simulink model "parallelizationTest"  (R2017a)
settings: Solver=FixedStepAuto  StartTime=0.0  StopTime=10  FixedStep=0.1  RelTol=1e-3
settings Model: Creator=TSu  LastModifiedBy=TSu
settings SolverCC: AutoInsertRateTranBlk=on
settings DebuggingCC: RootOutportRequireBusObject=error  StrictBusMsg=ErrorOnBusTreatedAsVector
settings HardwareCC: ProdBitPerLong=64  ProdBitPerPointer=32  ProdBitPerSizeT=32  ProdBitPerPtrDiffT=32  ProdLargestAtomicFloat=None  ProdHWDeviceType=Generic->Custom
settings SFSimCC: SimCustomHeaderCode="#include \"doubleIt.h\""  SimUserSources=doubleIt.c
settings RTWCC: PackageGeneratedCodeAndArtifacts=on  PackageName=testParallelization

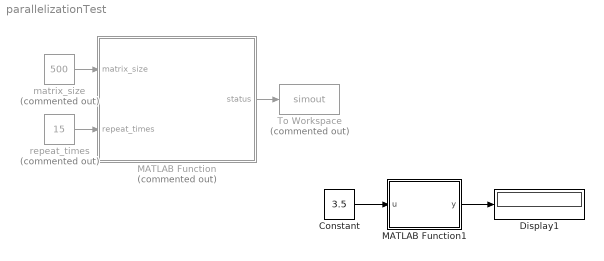
== system parallelizationTest ==
  Constant : Constant  Value=3.5
  Display1 : Display
  MATLAB Function : MATLAB Function  Commented=on  TreatAsAtomicUnit=on
  MATLAB Function1 : MATLAB Function  TreatAsAtomicUnit=on
  To Workspace : ToWorkspace  Commented=on  VariableName=simout  SaveFormat=Timeseries  SampleTime=-1
  matrix_size : Constant  Commented=on  Value=500
  repeat_times : Constant  Commented=on  Value=15
  wires:
  matrix_size/1 -> MATLAB Function/1(matrix_size)
  repeat_times/1 -> MATLAB Function/2(repeat_times)
  MATLAB Function/1(status) -> To Workspace/1
  Constant/1 -> MATLAB Function1/1(u)
  MATLAB Function1/1(y) -> Display1/1

== matlab function parallelizationTest/MATLAB Function1 ==
  data: u input; y output
function y = callingDoubleIt(u)
y = 0.0;
y = coder.ceval('doubleIt',u);

== matlab function parallelizationTest/MATLAB Function ==
  data: matrix_size input; status output; repeat_times input
function status = time_par_tests(matrix_size, repeat_times)
% time_par_tests: Perform a parallization test (baseline)

status = 0;
status = coder.ceval('time_par_tests',matrix_size, repeat_times);

end
